simulink model "RC_top_ACU"  (R2018b)
settings: Solver=VariableStepAuto  StartTime=0.0  StopTime=500000.0  RelTol=1e-3
libraries: simulink x4
(part 3 of 3)

== system RC_top_ACU/Global Model RC/ACU/C_steam_1/speed ==
  In1 : Inport
  In2 : Inport  Port=2
  EVAP_params : Inport  Port=3
  Coeff : Constant  Value=0.785
  Demux : Demux  Outputs=6
  Display : Display
  Display1 : Display
  Display2 : Display
  Divide : Product  Inputs=*/
  Divide1 : Product  Inputs=*/
  Product1 : Product  Inputs=4  SaturateOnIntegerOverflow=on  InputSameDT=on  OutDataTypeStr=Inherit: Same as first input
  Product13 : Product  SaturateOnIntegerOverflow=on  InputSameDT=on  OutDataTypeStr=Inherit: Same as first input
  Product2 : Product  Inputs=4  SaturateOnIntegerOverflow=on  InputSameDT=on  OutDataTypeStr=Inherit: Same as first input
  Product3 : Product  SaturateOnIntegerOverflow=on  InputSameDT=on  OutDataTypeStr=Inherit: Same as first input
  Product4 : Product  SaturateOnIntegerOverflow=on  InputSameDT=on  OutDataTypeStr=Inherit: Same as first input
  Sum : Sum  Inputs=++|
  T_0 : Constant  Value=273.15
  T_1 : Constant  Value=273.15
  T_2 : Constant  Value=0.003223135
  speed3 : Fcn  Expr=((0.003223135*(273+u))/24.69822264)/1.375
  Out1 : Outport
  wires:
  In1/1 -> Product3/1, Product13/1
  In2/1 -> Sum/1, speed3/1
  speed3/1 -> Product13/2
  EVAP_params/1 -> Demux/1
  Demux/2 -> Product1/2
  Demux/3 -> Product1/3
  Demux/4 -> Product1/4
  Sum/1 -> Product1/1
  T_0/1 -> Sum/2
  Demux/5 -> Product2/1
  Coeff/1 -> Product2/3
  T_1/1 -> Product2/4
  Product1/1 -> Divide/1
  Product2/1 -> Divide/2
  Divide/1 -> Divide1/1
  Demux/1 -> Divide1/2
  Divide1/1 -> Product3/2
  Demux/6 -> Product4/2, Product4/1
  Product4/1 -> Product2/2
  Product3/1 -> Out1/1, Display/1
  Product13/1 -> Display1/1
  T_2/1 -> Display2/1

== system RC_top_ACU/Global Model RC/ACU/C_steam_2/k1 ==
  In1 : Inport
  In2 : Inport  Port=2
  EVAP_params1 : Inport  Port=3
  Coeff : Constant  Value=0.785
  Demux : Demux  Outputs=6
  Display : Display
  Display1 : Display
  Display2 : Display
  Divide : Product  Inputs=*/
  Divide1 : Product  Inputs=*/
  Product1 : Product  Inputs=4  SaturateOnIntegerOverflow=on  InputSameDT=on  OutDataTypeStr=Inherit: Same as first input
  Product13 : Product  SaturateOnIntegerOverflow=on  InputSameDT=on  OutDataTypeStr=Inherit: Same as first input
  Product2 : Product  Inputs=4  SaturateOnIntegerOverflow=on  InputSameDT=on  OutDataTypeStr=Inherit: Same as first input
  Product3 : Product  SaturateOnIntegerOverflow=on  InputSameDT=on  OutDataTypeStr=Inherit: Same as first input
  Product4 : Product  SaturateOnIntegerOverflow=on  InputSameDT=on  OutDataTypeStr=Inherit: Same as first input
  Sum : Sum  Inputs=++|
  Sum1 : Sum  Inputs=|+-
  T_0 : Constant  Value=273.15
  T_1 : Constant  Value=273.15
  T_2 : Constant  Value=0.0000216487318
  T_3 : Constant  Value=0.003223135
  speed3 : Fcn  Expr=((0.003223135*(273+u))/24.69822264)/1.375-0.004302
  Out1 : Outport
  wires:
  speed3/1 -> Product13/1
  T_1/1 -> Product2/4
  Divide/1 -> Divide1/1
  EVAP_params1/1 -> Demux/1
  Demux/1 -> Divide1/2
  Demux/6 -> Product4/2, Product4/1
  In2/1 -> Product3/1, Product13/2
  Coeff/1 -> Product2/3
  In1/1 -> Sum/1, speed3/1
  Demux/4 -> Product1/4
  Demux/5 -> Product2/1
  Demux/3 -> Product1/3
  Product4/1 -> Product2/2
  Product3/1 -> Out1/1, Display/1
  T_0/1 -> Sum/2
  Product1/1 -> Divide/1
  Sum/1 -> Product1/1
  Demux/2 -> Product1/2
  Product13/1 -> Display1/1
  Sum1/1 -> Product3/2
  Divide1/1 -> Sum1/1
  T_2/1 -> Sum1/2
  T_3/1 -> Display2/1
  Product2/1 -> Divide/2

== system RC_top_ACU/Global Model RC/ACU/C_steam_2/speed ==
  In1 : Inport
  In2 : Inport  Port=2
  EVAP_params : Inport  Port=3
  Coeff : Constant  Value=0.785
  Demux : Demux  Outputs=6
  Display : Display
  Display1 : Display
  Display2 : Display
  Divide : Product  Inputs=*/
  Divide1 : Product  Inputs=*/
  Product1 : Product  Inputs=4  SaturateOnIntegerOverflow=on  InputSameDT=on  OutDataTypeStr=Inherit: Same as first input
  Product13 : Product  SaturateOnIntegerOverflow=on  InputSameDT=on  OutDataTypeStr=Inherit: Same as first input
  Product2 : Product  Inputs=4  SaturateOnIntegerOverflow=on  InputSameDT=on  OutDataTypeStr=Inherit: Same as first input
  Product3 : Product  SaturateOnIntegerOverflow=on  InputSameDT=on  OutDataTypeStr=Inherit: Same as first input
  Product4 : Product  SaturateOnIntegerOverflow=on  InputSameDT=on  OutDataTypeStr=Inherit: Same as first input
  Sum : Sum  Inputs=++|
  T_0 : Constant  Value=273.15
  T_1 : Constant  Value=273.15
  T_2 : Constant  Value=0.003223135
  speed3 : Fcn  Expr=((0.003223135*(273+u))/24.69822264)/1.375
  Out1 : Outport
  wires:
  In1/1 -> Product3/1, Product13/1
  In2/1 -> Sum/1, speed3/1
  speed3/1 -> Product13/2
  EVAP_params/1 -> Demux/1
  Demux/2 -> Product1/2
  Demux/3 -> Product1/3
  Demux/4 -> Product1/4
  Sum/1 -> Product1/1
  T_0/1 -> Sum/2
  Demux/5 -> Product2/1
  Coeff/1 -> Product2/3
  T_1/1 -> Product2/4
  Product1/1 -> Divide/1
  Product2/1 -> Divide/2
  Divide/1 -> Divide1/1
  Demux/1 -> Divide1/2
  Divide1/1 -> Product3/2
  Demux/6 -> Product4/2, Product4/1
  Product4/1 -> Product2/2
  Product3/1 -> Out1/1, Display/1
  Product13/1 -> Display1/1
  T_2/1 -> Display2/1

== system RC_top_ACU/Global Model RC/ACU/C_steam_3/k1 ==
  In1 : Inport
  In2 : Inport  Port=2
  EVAP_params1 : Inport  Port=3
  Coeff : Constant  Value=0.785
  Demux : Demux  Outputs=6
  Display : Display
  Display1 : Display
  Display2 : Display
  Divide : Product  Inputs=*/
  Divide1 : Product  Inputs=*/
  Product1 : Product  Inputs=4  SaturateOnIntegerOverflow=on  InputSameDT=on  OutDataTypeStr=Inherit: Same as first input
  Product13 : Product  SaturateOnIntegerOverflow=on  InputSameDT=on  OutDataTypeStr=Inherit: Same as first input
  Product2 : Product  Inputs=4  SaturateOnIntegerOverflow=on  InputSameDT=on  OutDataTypeStr=Inherit: Same as first input
  Product3 : Product  SaturateOnIntegerOverflow=on  InputSameDT=on  OutDataTypeStr=Inherit: Same as first input
  Product4 : Product  SaturateOnIntegerOverflow=on  InputSameDT=on  OutDataTypeStr=Inherit: Same as first input
  Sum : Sum  Inputs=++|
  Sum1 : Sum  Inputs=|+-
  T_0 : Constant  Value=273.15
  T_1 : Constant  Value=273.15
  T_2 : Constant  Value=0.0000216487318
  T_3 : Constant  Value=0.003223135
  speed3 : Fcn  Expr=((0.003223135*(273+u))/24.69822264)/1.375-0.004302
  Out1 : Outport
  wires:
  speed3/1 -> Product13/1
  T_1/1 -> Product2/4
  Divide/1 -> Divide1/1
  EVAP_params1/1 -> Demux/1
  Demux/1 -> Divide1/2
  Demux/6 -> Product4/2, Product4/1
  In2/1 -> Product3/1, Product13/2
  Coeff/1 -> Product2/3
  In1/1 -> Sum/1, speed3/1
  Demux/4 -> Product1/4
  Demux/5 -> Product2/1
  Demux/3 -> Product1/3
  Product4/1 -> Product2/2
  Product3/1 -> Out1/1, Display/1
  T_0/1 -> Sum/2
  Product1/1 -> Divide/1
  Sum/1 -> Product1/1
  Demux/2 -> Product1/2
  Product13/1 -> Display1/1
  Sum1/1 -> Product3/2
  Divide1/1 -> Sum1/1
  T_2/1 -> Sum1/2
  T_3/1 -> Display2/1
  Product2/1 -> Divide/2

== system RC_top_ACU/Global Model RC/ACU/C_steam_3/speed ==
  In1 : Inport
  In2 : Inport  Port=2
  EVAP_params : Inport  Port=3
  Coeff : Constant  Value=0.785
  Demux : Demux  Outputs=6
  Display : Display
  Display1 : Display
  Display2 : Display
  Divide : Product  Inputs=*/
  Divide1 : Product  Inputs=*/
  Product1 : Product  Inputs=4  SaturateOnIntegerOverflow=on  InputSameDT=on  OutDataTypeStr=Inherit: Same as first input
  Product13 : Product  SaturateOnIntegerOverflow=on  InputSameDT=on  OutDataTypeStr=Inherit: Same as first input
  Product2 : Product  Inputs=4  SaturateOnIntegerOverflow=on  InputSameDT=on  OutDataTypeStr=Inherit: Same as first input
  Product3 : Product  SaturateOnIntegerOverflow=on  InputSameDT=on  OutDataTypeStr=Inherit: Same as first input
  Product4 : Product  SaturateOnIntegerOverflow=on  InputSameDT=on  OutDataTypeStr=Inherit: Same as first input
  Sum : Sum  Inputs=++|
  T_0 : Constant  Value=273.15
  T_1 : Constant  Value=273.15
  T_2 : Constant  Value=0.003223135
  speed3 : Fcn  Expr=((0.003223135*(273+u))/24.69822264)/1.375
  Out1 : Outport
  wires:
  In1/1 -> Product3/1, Product13/1
  In2/1 -> Sum/1, speed3/1
  speed3/1 -> Product13/2
  EVAP_params/1 -> Demux/1
  Demux/2 -> Product1/2
  Demux/3 -> Product1/3
  Demux/4 -> Product1/4
  Sum/1 -> Product1/1
  T_0/1 -> Sum/2
  Demux/5 -> Product2/1
  Coeff/1 -> Product2/3
  T_1/1 -> Product2/4
  Product1/1 -> Divide/1
  Product2/1 -> Divide/2
  Divide/1 -> Divide1/1
  Demux/1 -> Divide1/2
  Divide1/1 -> Product3/2
  Demux/6 -> Product4/2, Product4/1
  Product4/1 -> Product2/2
  Product3/1 -> Out1/1, Display/1
  Product13/1 -> Display1/1
  T_2/1 -> Display2/1

== system RC_top_ACU/Global Model RC/ACU/C_steam_4/k1 ==
  In1 : Inport
  In2 : Inport  Port=2
  EVAP_params1 : Inport  Port=3
  Coeff : Constant  Value=0.785
  Demux : Demux  Outputs=6
  Display : Display
  Display1 : Display
  Display2 : Display
  Divide : Product  Inputs=*/
  Divide1 : Product  Inputs=*/
  Product1 : Product  Inputs=4  SaturateOnIntegerOverflow=on  InputSameDT=on  OutDataTypeStr=Inherit: Same as first input
  Product13 : Product  SaturateOnIntegerOverflow=on  InputSameDT=on  OutDataTypeStr=Inherit: Same as first input
  Product2 : Product  Inputs=4  SaturateOnIntegerOverflow=on  InputSameDT=on  OutDataTypeStr=Inherit: Same as first input
  Product3 : Product  SaturateOnIntegerOverflow=on  InputSameDT=on  OutDataTypeStr=Inherit: Same as first input
  Product4 : Product  SaturateOnIntegerOverflow=on  InputSameDT=on  OutDataTypeStr=Inherit: Same as first input
  Sum : Sum  Inputs=++|
  Sum1 : Sum  Inputs=|+-
  T_0 : Constant  Value=273.15
  T_1 : Constant  Value=273.15
  T_2 : Constant  Value=0.0000216487318
  T_3 : Constant  Value=0.003223135
  speed3 : Fcn  Expr=((0.003223135*(273+u))/24.69822264)/1.375-0.004302
  Out1 : Outport
  wires:
  speed3/1 -> Product13/1
  T_1/1 -> Product2/4
  Divide/1 -> Divide1/1
  EVAP_params1/1 -> Demux/1
  Demux/1 -> Divide1/2
  Demux/6 -> Product4/2, Product4/1
  In2/1 -> Product3/1, Product13/2
  Coeff/1 -> Product2/3
  In1/1 -> Sum/1, speed3/1
  Demux/4 -> Product1/4
  Demux/5 -> Product2/1
  Demux/3 -> Product1/3
  Product4/1 -> Product2/2
  Product3/1 -> Out1/1, Display/1
  T_0/1 -> Sum/2
  Product1/1 -> Divide/1
  Sum/1 -> Product1/1
  Demux/2 -> Product1/2
  Product13/1 -> Display1/1
  Sum1/1 -> Product3/2
  Divide1/1 -> Sum1/1
  T_2/1 -> Sum1/2
  T_3/1 -> Display2/1
  Product2/1 -> Divide/2

== system RC_top_ACU/Global Model RC/ACU/C_steam_4/speed ==
  In1 : Inport
  In2 : Inport  Port=2
  EVAP_params : Inport  Port=3
  Coeff : Constant  Value=0.785
  Demux : Demux  Outputs=6
  Display : Display
  Display1 : Display
  Display2 : Display
  Divide : Product  Inputs=*/
  Divide1 : Product  Inputs=*/
  Product1 : Product  Inputs=4  SaturateOnIntegerOverflow=on  InputSameDT=on  OutDataTypeStr=Inherit: Same as first input
  Product13 : Product  SaturateOnIntegerOverflow=on  InputSameDT=on  OutDataTypeStr=Inherit: Same as first input
  Product2 : Product  Inputs=4  SaturateOnIntegerOverflow=on  InputSameDT=on  OutDataTypeStr=Inherit: Same as first input
  Product3 : Product  SaturateOnIntegerOverflow=on  InputSameDT=on  OutDataTypeStr=Inherit: Same as first input
  Product4 : Product  SaturateOnIntegerOverflow=on  InputSameDT=on  OutDataTypeStr=Inherit: Same as first input
  Sum : Sum  Inputs=++|
  T_0 : Constant  Value=273.15
  T_1 : Constant  Value=273.15
  T_2 : Constant  Value=0.003223135
  speed3 : Fcn  Expr=((0.003223135*(273+u))/24.69822264)/1.375
  Out1 : Outport
  wires:
  In1/1 -> Product3/1, Product13/1
  In2/1 -> Sum/1, speed3/1
  speed3/1 -> Product13/2
  EVAP_params/1 -> Demux/1
  Demux/2 -> Product1/2
  Demux/3 -> Product1/3
  Demux/4 -> Product1/4
  Sum/1 -> Product1/1
  T_0/1 -> Sum/2
  Demux/5 -> Product2/1
  Coeff/1 -> Product2/3
  T_1/1 -> Product2/4
  Product1/1 -> Divide/1
  Product2/1 -> Divide/2
  Divide/1 -> Divide1/1
  Demux/1 -> Divide1/2
  Divide1/1 -> Product3/2
  Demux/6 -> Product4/2, Product4/1
  Product4/1 -> Product2/2
  Product3/1 -> Out1/1, Display/1
  Product13/1 -> Display1/1
  T_2/1 -> Display2/1

== system RC_top_ACU/Global Model RC/ACU/Subsystem/Pr.f ==
  In1 : Inport
  1/T : Gain
  Fcn : Fcn  Expr=(u/0.152)^(1/2)
  Gain1 : Gain
  "Gf, kmol/h1" : Display
  "Gf, kmol/h2" : Display
  Integrator : Integrator  InitialCondition=403.6
  Sum1 : Sum
  Sum2 : Sum  Inputs=-+
  U1 : Constant  Value=380
  kn : Gain  Gain=4300
  Out1 : Outport
  wires:
  kn/1 -> 1/T/1, Gain1/1
  1/T/1 -> Integrator/1, "Gf, kmol/h1"/1
  Integrator/1 -> Sum1/2, "Gf, kmol/h2"/1
  Gain1/1 -> Sum1/1
  Sum1/1 -> Sum2/2
  U1/1 -> Sum2/1
  In1/1 -> kn/1
  Fcn/1 -> Out1/1
  Sum2/1 -> Fcn/1

== system RC_top_ACU/Global Model RC/ACU/Subsystem/SbS RASCHET G ==
  In1 : Inport
  In2 : Inport  Port=2
  In3 : Inport  Port=3
  In4 : Inport  Port=4
  "Cd, mol.dol" : Fcn  Expr=(u/18.02)/((u/18.02)+((1-u)/106.12))
  "Cna, mol.dol" : Fcn  Expr=(u/18.02)/((u/18.02)+((1-u)/106.12))
  "Cra, mol.dol" : Fcn  Expr=(u/18.02)/((u/18.02)+((1-u)/106.12))
  Fcn1 : Fcn  Expr=1/u
  Fcn10 : Fcn  Expr=1/u
  Fcn6 : Fcn  Expr=1/u
  Gd*(R+1) : Fcn  Expr=u*(0.5+1)
  Gd*R : Fcn  Expr=u*0.5
  "Md, kg/kmol" : Fcn  Expr=18.02*u+106.12*(1-u)
  "Mna, kg/kmol1" : Fcn  Expr=18.02*u+106.12*(1-u)
  "Mra, kg/kmol" : Fcn  Expr=18.02*u+106.12*(1-u)
  Pr{,1..8} (9 alike) : Product  RndMeth=Zero
  Sbtr2 : Sum  Inputs=+-
  Sbtr3 : Sum  Inputs=-+
  Str : Sum  Inputs=-+
  Str1 : Sum  Inputs=-+
  Out1 : Outport
  Out2 : Outport  Port=2
  Out3 : Outport  Port=3
  Out4 : Outport  Port=4
  Out5 : Outport  Port=5
  Out6 : Outport  Port=6
  Out7 : Outport  Port=7
  Out8 : Outport  Port=8
  Out9 : Outport  Port=9
  wires:
  "Mna, kg/kmol1"/1 -> Pr3/1
  "Cna, mol.dol"/1 -> "Mna, kg/kmol1"/1, Str/1, Sbtr3/1, Sbtr2/1
  "Cra, mol.dol"/1 -> "Mra, kg/kmol"/1, Str1/1, Sbtr3/2
  "Cd, mol.dol"/1 -> "Md, kg/kmol"/1, Str1/2, Str/2, Sbtr2/2
  "Mra, kg/kmol"/1 -> Fcn6/1
  Fcn6/1 -> Pr/2
  Pr/1 -> Pr2/1, Out3/1, Pr5/1
  Str/1 -> Fcn10/1
  Fcn10/1 -> Pr1/2
  Pr2/1 -> Pr3/2, Out2/1
  Pr1/1 -> Pr2/2
  Str1/1 -> Pr1/1
  Fcn1/1 -> Pr4/2
  Pr5/1 -> Pr6/1, Gd*(R+1)/1, Gd*R/1, Out4/1
  Pr4/1 -> Pr5/2
  "Md, kg/kmol"/1 -> Pr6/2, Pr7/2, Pr8/2
  Sbtr2/1 -> Fcn1/1
  Sbtr3/1 -> Pr4/1
  Gd*(R+1)/1 -> Pr7/1, Out6/1
  Gd*R/1 -> Pr8/1, Out8/1
  In1/1 -> "Cna, mol.dol"/1
  Pr3/1 -> Out1/1
  In2/1 -> Pr/1
  In3/1 -> "Cra, mol.dol"/1
  Pr6/1 -> Out5/1
  In4/1 -> "Cd, mol.dol"/1
  Pr7/1 -> Out7/1
  Pr8/1 -> Out9/1

== system RC_top_ACU/Global Model RC/ACU/АВО/Pr.f ==
  In1 : Inport
  1/T : Gain
  Fcn : Fcn  Expr=(u/0.152)^(1/2)
  Gain1 : Gain
  "Gf, kmol/h1" : Display
  "Gf, kmol/h2" : Display
  Integrator : Integrator  InitialCondition=403.6
  Sum1 : Sum
  Sum2 : Sum  Inputs=-+
  U1 : Constant  Value=380
  kn : Gain  Gain=4300
  Out1 : Outport
  wires:
  kn/1 -> 1/T/1, Gain1/1
  1/T/1 -> Integrator/1, "Gf, kmol/h1"/1
  Integrator/1 -> Sum1/2, "Gf, kmol/h2"/1
  Gain1/1 -> Sum1/1
  Sum1/1 -> Sum2/2
  U1/1 -> Sum2/1
  In1/1 -> kn/1
  Fcn/1 -> Out1/1
  Sum2/1 -> Fcn/1

== system RC_top_ACU/Global Model RC/ACU/АВО/SbS RASCHET G ==
  In1 : Inport
  In2 : Inport  Port=2
  In3 : Inport  Port=3
  In4 : Inport  Port=4
  "Cd, mol.dol" : Fcn  Expr=(u/18.02)/((u/18.02)+((1-u)/106.12))
  "Cna, mol.dol" : Fcn  Expr=(u/18.02)/((u/18.02)+((1-u)/106.12))
  "Cra, mol.dol" : Fcn  Expr=(u/18.02)/((u/18.02)+((1-u)/106.12))
  Fcn1 : Fcn  Expr=1/u
  Fcn10 : Fcn  Expr=1/u
  Fcn6 : Fcn  Expr=1/u
  Gd*(R+1) : Fcn  Expr=u*(0.5+1)
  Gd*R : Fcn  Expr=u*0.5
  "Md, kg/kmol" : Fcn  Expr=18.02*u+106.12*(1-u)
  "Mna, kg/kmol1" : Fcn  Expr=18.02*u+106.12*(1-u)
  "Mra, kg/kmol" : Fcn  Expr=18.02*u+106.12*(1-u)
  Pr{,1..8} (9 alike) : Product  RndMeth=Zero
  Sbtr2 : Sum  Inputs=+-
  Sbtr3 : Sum  Inputs=-+
  Str : Sum  Inputs=-+
  Str1 : Sum  Inputs=-+
  Out1 : Outport
  Out2 : Outport  Port=2
  Out3 : Outport  Port=3
  Out4 : Outport  Port=4
  Out5 : Outport  Port=5
  Out6 : Outport  Port=6
  Out7 : Outport  Port=7
  Out8 : Outport  Port=8
  Out9 : Outport  Port=9
  wires:
  "Mna, kg/kmol1"/1 -> Pr3/1
  "Cna, mol.dol"/1 -> "Mna, kg/kmol1"/1, Str/1, Sbtr3/1, Sbtr2/1
  "Cra, mol.dol"/1 -> "Mra, kg/kmol"/1, Str1/1, Sbtr3/2
  "Cd, mol.dol"/1 -> "Md, kg/kmol"/1, Str1/2, Str/2, Sbtr2/2
  "Mra, kg/kmol"/1 -> Fcn6/1
  Fcn6/1 -> Pr/2
  Pr/1 -> Pr2/1, Out3/1, Pr5/1
  Str/1 -> Fcn10/1
  Fcn10/1 -> Pr1/2
  Pr2/1 -> Pr3/2, Out2/1
  Pr1/1 -> Pr2/2
  Str1/1 -> Pr1/1
  Fcn1/1 -> Pr4/2
  Pr5/1 -> Pr6/1, Gd*(R+1)/1, Gd*R/1, Out4/1
  Pr4/1 -> Pr5/2
  "Md, kg/kmol"/1 -> Pr6/2, Pr7/2, Pr8/2
  Sbtr2/1 -> Fcn1/1
  Sbtr3/1 -> Pr4/1
  Gd*(R+1)/1 -> Pr7/1, Out6/1
  Gd*R/1 -> Pr8/1, Out8/1
  In1/1 -> "Cna, mol.dol"/1
  Pr3/1 -> Out1/1
  In2/1 -> Pr/1
  In3/1 -> "Cra, mol.dol"/1
  Pr6/1 -> Out5/1
  In4/1 -> "Cd, mol.dol"/1
  Pr7/1 -> Out7/1
  Pr8/1 -> Out9/1

== system RC_top_ACU/Global Model RC/FULL_RC_1/АВО1/Pr.f ==
  In1 : Inport
  1/T : Gain
  Fcn : Fcn  Expr=(u/0.152)^(1/2)
  Gain1 : Gain
  "Gf, kmol/h1" : Display
  "Gf, kmol/h2" : Display
  Integrator : Integrator  InitialCondition=403.6
  Sum1 : Sum
  Sum2 : Sum  Inputs=-+
  U1 : Constant  Value=380
  kn : Gain  Gain=4300
  Out1 : Outport
  wires:
  kn/1 -> 1/T/1, Gain1/1
  1/T/1 -> Integrator/1, "Gf, kmol/h1"/1
  Integrator/1 -> Sum1/2, "Gf, kmol/h2"/1
  Gain1/1 -> Sum1/1
  Sum1/1 -> Sum2/2
  U1/1 -> Sum2/1
  In1/1 -> kn/1
  Fcn/1 -> Out1/1
  Sum2/1 -> Fcn/1

== system RC_top_ACU/Global Model RC/FULL_RC_1/АВО1/SbS RASCHET G ==
  In1 : Inport
  In2 : Inport  Port=2
  In3 : Inport  Port=3
  In4 : Inport  Port=4
  "Cd, mol.dol" : Fcn  Expr=(u/18.02)/((u/18.02)+((1-u)/106.12))
  "Cna, mol.dol" : Fcn  Expr=(u/18.02)/((u/18.02)+((1-u)/106.12))
  "Cra, mol.dol" : Fcn  Expr=(u/18.02)/((u/18.02)+((1-u)/106.12))
  Fcn1 : Fcn  Expr=1/u
  Fcn10 : Fcn  Expr=1/u
  Fcn6 : Fcn  Expr=1/u
  Gd*(R+1) : Fcn  Expr=u*(0.5+1)
  Gd*R : Fcn  Expr=u*0.5
  "Md, kg/kmol" : Fcn  Expr=18.02*u+106.12*(1-u)
  "Mna, kg/kmol1" : Fcn  Expr=18.02*u+106.12*(1-u)
  "Mra, kg/kmol" : Fcn  Expr=18.02*u+106.12*(1-u)
  Pr{,1..8} (9 alike) : Product  RndMeth=Zero
  Sbtr2 : Sum  Inputs=+-
  Sbtr3 : Sum  Inputs=-+
  Str : Sum  Inputs=-+
  Str1 : Sum  Inputs=-+
  Out1 : Outport
  Out2 : Outport  Port=2
  Out3 : Outport  Port=3
  Out4 : Outport  Port=4
  Out5 : Outport  Port=5
  Out6 : Outport  Port=6
  Out7 : Outport  Port=7
  Out8 : Outport  Port=8
  Out9 : Outport  Port=9
  wires:
  "Mna, kg/kmol1"/1 -> Pr3/1
  "Cna, mol.dol"/1 -> "Mna, kg/kmol1"/1, Str/1, Sbtr3/1, Sbtr2/1
  "Cra, mol.dol"/1 -> "Mra, kg/kmol"/1, Str1/1, Sbtr3/2
  "Cd, mol.dol"/1 -> "Md, kg/kmol"/1, Str1/2, Str/2, Sbtr2/2
  "Mra, kg/kmol"/1 -> Fcn6/1
  Fcn6/1 -> Pr/2
  Pr/1 -> Pr2/1, Out3/1, Pr5/1
  Str/1 -> Fcn10/1
  Fcn10/1 -> Pr1/2
  Pr2/1 -> Pr3/2, Out2/1
  Pr1/1 -> Pr2/2
  Str1/1 -> Pr1/1
  Fcn1/1 -> Pr4/2
  Pr5/1 -> Pr6/1, Gd*(R+1)/1, Gd*R/1, Out4/1
  Pr4/1 -> Pr5/2
  "Md, kg/kmol"/1 -> Pr6/2, Pr7/2, Pr8/2
  Sbtr2/1 -> Fcn1/1
  Sbtr3/1 -> Pr4/1
  Gd*(R+1)/1 -> Pr7/1, Out6/1
  Gd*R/1 -> Pr8/1, Out8/1
  In1/1 -> "Cna, mol.dol"/1
  Pr3/1 -> Out1/1
  In2/1 -> Pr/1
  In3/1 -> "Cra, mol.dol"/1
  Pr6/1 -> Out5/1
  In4/1 -> "Cd, mol.dol"/1
  Pr7/1 -> Out7/1
  Pr8/1 -> Out9/1

== system RC_top_ACU/Global Model RC/FULL_RC_2/AWC/Pr.f ==
  In1 : Inport
  1/T : Gain
  Fcn : Fcn  Expr=(u/0.152)^(1/2)
  Gain1 : Gain
  "Gf, kmol/h1" : Display
  "Gf, kmol/h2" : Display
  Integrator : Integrator  InitialCondition=403.6
  Sum1 : Sum
  Sum2 : Sum  Inputs=-+
  U1 : Constant  Value=380
  kn : Gain  Gain=4300
  Out1 : Outport
  wires:
  kn/1 -> 1/T/1, Gain1/1
  1/T/1 -> Integrator/1, "Gf, kmol/h1"/1
  Integrator/1 -> Sum1/2, "Gf, kmol/h2"/1
  Gain1/1 -> Sum1/1
  Sum1/1 -> Sum2/2
  U1/1 -> Sum2/1
  In1/1 -> kn/1
  Fcn/1 -> Out1/1
  Sum2/1 -> Fcn/1

== system RC_top_ACU/Global Model RC/FULL_RC_2/G()/SbS RASCHET G ==
  In1 : Inport
  In2 : Inport  Port=2
  In3 : Inport  Port=3
  In4 : Inport  Port=4
  "Cd, mol.dol" : Fcn  Expr=(u/18.02)/((u/18.02)+((1-u)/106.12))
  "Cna, mol.dol" : Fcn  Expr=(u/18.02)/((u/18.02)+((1-u)/106.12))
  "Cra, mol.dol" : Fcn  Expr=(u/18.02)/((u/18.02)+((1-u)/106.12))
  Fcn1 : Fcn  Expr=1/u
  Fcn10 : Fcn  Expr=1/u
  Fcn6 : Fcn  Expr=1/u
  Gd*(R+1) : Fcn  Expr=u*(0.5+1)
  Gd*R : Fcn  Expr=u*0.5
  "Md, kg/kmol" : Fcn  Expr=18.02*u+106.12*(1-u)
  "Mna, kg/kmol1" : Fcn  Expr=18.02*u+106.12*(1-u)
  "Mra, kg/kmol" : Fcn  Expr=18.02*u+106.12*(1-u)
  Pr{,1..8} (9 alike) : Product  RndMeth=Zero
  Sbtr2 : Sum  Inputs=+-
  Sbtr3 : Sum  Inputs=-+
  Str : Sum  Inputs=-+
  Str1 : Sum  Inputs=-+
  Out1 : Outport
  Out2 : Outport  Port=2
  Out3 : Outport  Port=3
  Out4 : Outport  Port=4
  Out5 : Outport  Port=5
  Out6 : Outport  Port=6
  Out7 : Outport  Port=7
  Out8 : Outport  Port=8
  Out9 : Outport  Port=9
  wires:
  "Mna, kg/kmol1"/1 -> Pr3/1
  "Cna, mol.dol"/1 -> "Mna, kg/kmol1"/1, Str/1, Sbtr3/1, Sbtr2/1
  "Cra, mol.dol"/1 -> "Mra, kg/kmol"/1, Str1/1, Sbtr3/2
  "Cd, mol.dol"/1 -> "Md, kg/kmol"/1, Str1/2, Str/2, Sbtr2/2
  "Mra, kg/kmol"/1 -> Fcn6/1
  Fcn6/1 -> Pr/2
  Pr/1 -> Pr2/1, Out3/1, Pr5/1
  Str/1 -> Fcn10/1
  Fcn10/1 -> Pr1/2
  Pr2/1 -> Out2/1, Pr3/2
  Pr1/1 -> Pr2/2
  Str1/1 -> Pr1/1
  Fcn1/1 -> Pr4/2
  Pr5/1 -> Pr6/1, Gd*(R+1)/1, Gd*R/1, Out4/1
  Pr4/1 -> Pr5/2
  "Md, kg/kmol"/1 -> Pr6/2, Pr7/2, Pr8/2
  Sbtr2/1 -> Fcn1/1
  Sbtr3/1 -> Pr4/1
  Gd*(R+1)/1 -> Pr7/1, Out6/1
  Gd*R/1 -> Pr8/1, Out8/1
  In1/1 -> "Cna, mol.dol"/1
  Pr3/1 -> Out1/1
  In2/1 -> Pr/1
  In3/1 -> "Cra, mol.dol"/1
  Pr6/1 -> Out5/1
  In4/1 -> "Cd, mol.dol"/1
  Pr7/1 -> Out7/1
  Pr8/1 -> Out9/1

== system RC_top_ACU/Global Model RC/RC_top/C_steam_1/k1 ==
  In1 : Inport
  In2 : Inport  Port=2
  Product13 : Product  SaturateOnIntegerOverflow=on  InputSameDT=on  OutDataTypeStr=Inherit: Same as first input
  speed3 : Fcn  Expr=((0.003223135*(273+u))/24.69822264)/0.5-0.0000216487318
  Out1 : Outport
  wires:
  Product13/1 -> Out1/1
  speed3/1 -> Product13/1
  In1/1 -> speed3/1
  In2/1 -> Product13/2

== system RC_top_ACU/Global Model RC/RC_top/C_steam_1/speed ==
  In1 : Inport
  In2 : Inport  Port=2
  Product13 : Product  SaturateOnIntegerOverflow=on  InputSameDT=on  OutDataTypeStr=Inherit: Same as first input
  speed3 : Fcn  Expr=((0.003223135*(273+u))/24.69822264)/0.5
  Out1 : Outport
  wires:
  In1/1 -> Product13/1
  In2/1 -> speed3/1
  speed3/1 -> Product13/2
  Product13/1 -> Out1/1

== system RC_top_ACU/Global Model RC/RC_top/C_steam_2/k1 ==
  In1 : Inport
  In2 : Inport  Port=2
  Product13 : Product  SaturateOnIntegerOverflow=on  InputSameDT=on  OutDataTypeStr=Inherit: Same as first input
  speed3 : Fcn  Expr=((0.003223135*(273+u))/24.69822264)/0.5-0.004302
  Out1 : Outport
  wires:
  Product13/1 -> Out1/1
  speed3/1 -> Product13/1
  In1/1 -> speed3/1
  In2/1 -> Product13/2

== system RC_top_ACU/Global Model RC/RC_top/C_steam_2/speed ==
  In1 : Inport
  In2 : Inport  Port=2
  Product13 : Product  SaturateOnIntegerOverflow=on  InputSameDT=on  OutDataTypeStr=Inherit: Same as first input
  speed3 : Fcn  Expr=((0.003223135*(273+u))/24.69822264)/0.5
  Out1 : Outport
  wires:
  In1/1 -> Product13/1
  In2/1 -> speed3/1
  speed3/1 -> Product13/2
  Product13/1 -> Out1/1

== system RC_top_ACU/Global Model RC/RC_top/C_steam_3/k1 ==
  In1 : Inport
  In2 : Inport  Port=2
  Product13 : Product  SaturateOnIntegerOverflow=on  InputSameDT=on  OutDataTypeStr=Inherit: Same as first input
  speed3 : Fcn  Expr=((0.003223135*(273+u))/24.69822264)/0.5-0.004302
  Out1 : Outport
  wires:
  Product13/1 -> Out1/1
  speed3/1 -> Product13/1
  In1/1 -> speed3/1
  In2/1 -> Product13/2

== system RC_top_ACU/Global Model RC/RC_top/C_steam_3/speed ==
  In1 : Inport
  In2 : Inport  Port=2
  Product13 : Product  SaturateOnIntegerOverflow=on  InputSameDT=on  OutDataTypeStr=Inherit: Same as first input
  speed3 : Fcn  Expr=((0.003223135*(273+u))/24.69822264)/0.5
  Out1 : Outport
  wires:
  In1/1 -> Product13/1
  In2/1 -> speed3/1
  speed3/1 -> Product13/2
  Product13/1 -> Out1/1
